simulink library "LopesDevelopmentLibrary"  (R2015b)
settings: Solver=ode45  StartTime=0.0  StopTime=10.0  RelTol=1e-3
values from neighbouring files (symbols this model uses):
  d2r = @(d) d*(pi/180)    [LopesDevelopmentLibrary_LoadParameters.m]
  ts = LopesParams.ts    [LopesDevelopmentLibrary_LoadParameters.m]
undefined symbols (not defined in the file or in its folder): anyParameterChanged, DiscIntNeverNeededParam, gcbh, LHF, LKF, LopesParams, macaddr, mxpcnetworkconfig, mxpcrtudprx, mxpcrtudptx, patientParametersChanged, port, PX, PZ, RHF, RKF, SelectorLOPESInSize, StrideTime_s, Time
undefined symbols (not defined in the file): LopesParamsSendDataArrayLen
libraries: LopesDevelopmentLibrary x288, simulink x98, dspmtrx3 x47, xpciplib x6, xpcnetworkbufferlib x5, dspsigops x4, dspstat3 x3, xpcethernetlib x2, visionstatistics x2, xpcseriallib x2, nmc x1, simulink_extras x1
(part 6 of 12)

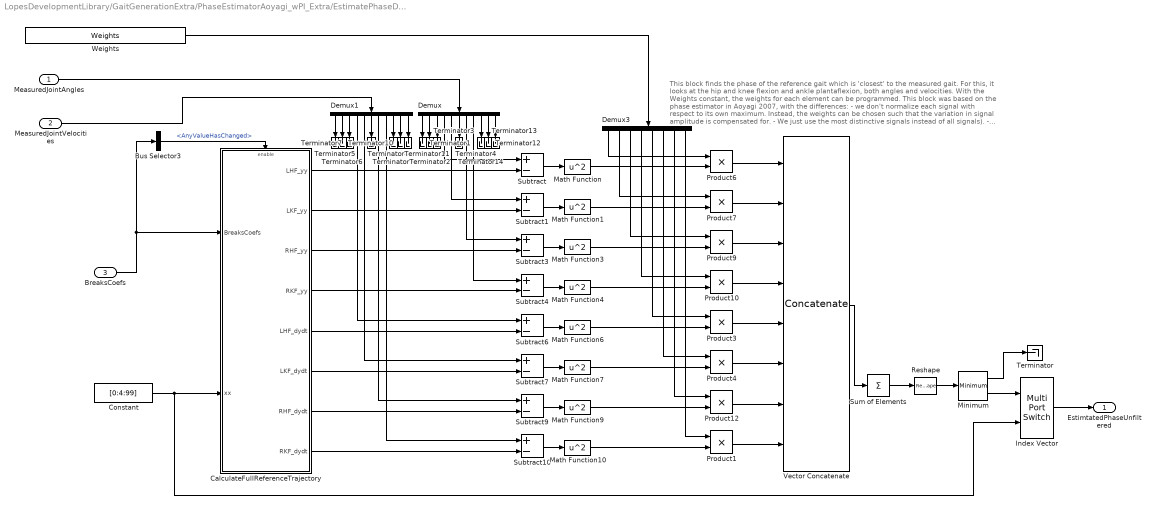
== system LopesDevelopmentLibrary/GaitGenerationExtra/PhaseEstimatorAoyagi_wPI_Extra/EstimatePhaseDirectlyAoyagi ==
  note: This block finds the phase of the reference gait which is 'closest' to the
      | measured gait. For this, it looks at the hip and knee flexion and ankle plantaflexion,
      | both angles and velocities. With the Weights constant, the weights for each element
      | can be programmed.
      | This block was based on the phase estimator in Aoyagi 2007, with the differences:
      | - we don't normalize each signal with respect to its own maximum. Instead, the weights
      | can be chosen such that the variation in signal amplitude is compensated for.
      | - We just use the most distinctive signals instead of all signals).
      | - The phase is expressed in percent  [0,100) instead of [0,1).
  MeasuredJointAngles : Inport
  MeasuredJointVelocities : Inport  Port=2
  BreaksCoefs : Inport  Port=3
  Bus Selector3 : BusSelector  OutputSignals=AnyValueHasChanged
  CalculateFullReferenceTrajectory : Subsystem
  Constant : Constant  Value=[0:4:99]
  Demux : Demux  Outputs=11
  Demux1 : Demux  Outputs=11
  Demux3 : Demux  Outputs=8
  Index Vector : MultiPortSwitch  Inputs=1
  Math Function{,1,3..4,6..7,9..10} (8 alike) : Math  Operator=square  SaturateOnIntegerOverflow=on
  Minimum : dspstat3/Minimum  fcn=Value and Index  reset=None  InputProcessing=Columns as channels (frame based)  indexBase=One  operateOver=Each column  Dimension=1  operation=minimum  roiEnable=off  roiType=Rectangles  roiPortion=Entire ROI  roiOutput=Individual statistics for each ROI  roiFlag=off  roundingMode=Floor  overflowMode=off
  Product{1,3..4,6..7,9..10,12} (8 alike) : Product  RndMeth=Zero
  Reshape : Reshape
  Subtract{,1,3..4,6..7,9..10} (8 alike) : Sum  Inputs=+-
  Sum of Elements : Sum  Inputs=+  CollapseMode=Specified dimension  CollapseDim=2
  Terminator{,1..14} (15 alike) : Terminator
  Vector Concatenate : Concatenate  NumInputs=8  Mode=Multidimensional array  ConcatenateDimension=2
  Weights : Constant  Value=Weights
  EstimtatedPhaseUnfiltered : Outport
  wires:
  Demux3/8 -> Product1/1
  Demux3/7 -> Product12/1
  Demux3/6 -> Product4/1
  Demux3/5 -> Product3/1
  Demux3/4 -> Product10/1
  Demux3/3 -> Product9/1
  Demux3/2 -> Product7/1
  Demux3/1 -> Product6/1
  Bus Selector3/1 -> CalculateFullReferenceTrajectory/Enable  "<AnyValueHasChanged>"
  CalculateFullReferenceTrajectory/8(RKF_dydt) -> Subtract10/2
  CalculateFullReferenceTrajectory/7(RHF_dydt) -> Subtract9/2
  CalculateFullReferenceTrajectory/6(LKF_dydt) -> Subtract7/2
  CalculateFullReferenceTrajectory/5(LHF_dydt) -> Subtract6/2
  CalculateFullReferenceTrajectory/4(RKF_yy) -> Subtract4/2
  CalculateFullReferenceTrajectory/3(RHF_yy) -> Subtract3/2
  CalculateFullReferenceTrajectory/2(LKF_yy) -> Subtract1/2
  CalculateFullReferenceTrajectory/1(LHF_yy) -> Subtract/2
  Reshape/1 -> Minimum/1
  Product1/1 -> Vector Concatenate/8
  Product12/1 -> Vector Concatenate/7
  Product3/1 -> Vector Concatenate/5
  Product4/1 -> Vector Concatenate/6
  Math Function10/1 -> Product1/2
  Math Function9/1 -> Product12/2
  Math Function7/1 -> Product4/2
  Math Function6/1 -> Product3/2
  Demux1/8 -> Subtract10/1
  Demux1/7 -> Subtract9/1
  Demux1/5 -> Subtract7/1
  Demux1/4 -> Subtract6/1
  Subtract10/1 -> Math Function10/1
  Subtract9/1 -> Math Function9/1
  Subtract7/1 -> Math Function7/1
  Subtract6/1 -> Math Function6/1
  MeasuredJointVelocities/1 -> Demux1/1
  Minimum/2 -> Index Vector/1
  Sum of Elements/1 -> Reshape/1
  Vector Concatenate/1 -> Sum of Elements/1
  Product10/1 -> Vector Concatenate/4
  Product9/1 -> Vector Concatenate/3
  Product6/1 -> Vector Concatenate/1
  Product7/1 -> Vector Concatenate/2
  Weights/1 -> Demux3/1
  Math Function4/1 -> Product10/2
  Math Function3/1 -> Product9/2
  Math Function1/1 -> Product7/2
  Math Function/1 -> Product6/2
  Subtract4/1 -> Math Function4/1
  Subtract3/1 -> Math Function3/1
  Subtract1/1 -> Math Function1/1
  Subtract/1 -> Math Function/1
  Demux/8 -> Subtract4/1
  Demux/7 -> Subtract3/1
  Index Vector/1 -> EstimtatedPhaseUnfiltered/1
  BreaksCoefs/1 -> CalculateFullReferenceTrajectory/1(BreaksCoefs), Bus Selector3/1
  MeasuredJointAngles/1 -> Demux/1
  Constant/1 -> CalculateFullReferenceTrajectory/2(xx), Index Vector/2
  Demux/4 -> Subtract/1
  Demux/5 -> Subtract1/1
  Minimum/1 -> Terminator/1
  Demux1/6 -> Terminator8/1
  Demux1/3 -> Terminator7/1
  Demux1/2 -> Terminator6/1
  Demux1/1 -> Terminator5/1
  Demux/1 -> Terminator1/1
  Demux/2 -> Terminator2/1
  Demux/3 -> Terminator3/1
  Demux/6 -> Terminator4/1
  Demux1/9 -> Terminator9/1
  Demux1/10 -> Terminator10/1
  Demux1/11 -> Terminator11/1
  Demux/11 -> Terminator13/1
  Demux/10 -> Terminator12/1
  Demux/9 -> Terminator14/1

== system LopesDevelopmentLibrary/GaitGenerationExtra/PhaseEstimatorAoyagi_wPI_Extra/PhaseFilterAoyagi ==
  note: This filter is based on the filter described in Aoyagi 2007.
      | It differs on the following points:
      | - Range [0,100) %, not [0,1) scale.
      | - Different implementation of wrap around integration (Aoyagi uses a resettable integrator; I use a mod 100)
      | - AoyagiFilterGain should be the same as in the paper (the error is 100 times larger than Aoyagi's, but so is
      |    the range of the integration). I found however that 2.5 for a gain [Aoyagi 2007] is quite low.
      | - In the figure in the paper no saturation is shown, but in the text they tell that there is saturation. I use it
      |    here too (so that phase cannot go backwards and cannot go rise too fast).
  note: "'PI-controller". Makes sure that the phase error will eventually
      | go to zero. Hopefully this will make the system better. However, the integral is
      | limited to -20..20 to prevent problems when a non-walking state is detected.
  EstimatedPhaseUnfiltered : Inport
  ReferenceStrideTime : Inport  Port=2
  ResetHighActive : Inport  Port=3
  x0 : Inport  Port=4
  FinalState : Inport  Port=5
  AoyagiFilterGain : Gain  Gain=AoyagiFilterGain
  CalculateStridesPerSec : Math  Operator=reciprocal  SaturateOnIntegerOverflow=on
  Compare To Constant : simulink/Logic and Bit Operations/Compare To Constant  relop=~=  const=1  OutDataTypeStr=boolean
  Divide : Product  Inputs=/*
  FinalStateFinisher : Subsystem
  Gain : Gain  Gain=3
  Gain1 : Gain  Gain=0.2
  IntegralTimeConstant : Constant  Value=AoyagiIntegralTimeConstant
  Integrator : Integrator  ExternalReset=level  InitialConditionSource=external
  Integrator1 : Integrator  ExternalReset=level  LimitOutput=on  UpperSaturationLimit=20  LowerSaturationLimit=-20
  PhaseWrapper : LopesDevelopmentLibrary/Various/PhaseWrapper
  Product : Product  OutDataTypeStr=double
  Saturation Dynamic : simulink/Discontinuities/Saturation Dynamic  OutMin=[]  OutMax=[]  OutDataTypeStr=Inherit: Same as second input  OutDataType=fixdt(1, 16)  OutScaling=2^-10  DoSatur=off
  Sum : Sum  Inputs=|+-
  Sum1 : Sum  Inputs=++|
  Sum2 : Sum  Inputs=++|
  ToPercentPerSec : Gain  Gain=100
  Wrap_Min50_Plus50 : Subsystem
  EstimatedPhase : Outport
  EstimatedPhaseRate : Outport  Port=2
  wires:
  ResetHighActive/1 -> Integrator1/2, Compare To Constant/1, Integrator/2
  Integrator/1 -> PhaseWrapper/1
  EstimatedPhaseUnfiltered/1 -> Sum/1
  Sum1/1 -> Saturation Dynamic/2
  AoyagiFilterGain/1 -> Sum1/2, Divide/2
  ToPercentPerSec/1 -> Sum2/2, Gain1/1, Gain/1
  PhaseWrapper/1 -> EstimatedPhase/1, Sum/2
  CalculateStridesPerSec/1 -> ToPercentPerSec/1
  Wrap_Min50_Plus50/1(Out) -> AoyagiFilterGain/1
  Sum/1 -> Wrap_Min50_Plus50/1(In)
  ReferenceStrideTime/1 -> CalculateStridesPerSec/1
  Gain1/1 -> Saturation Dynamic/3
  Gain/1 -> Saturation Dynamic/1
  IntegralTimeConstant/1 -> Divide/1
  Divide/1 -> Integrator1/1
  Integrator1/1 -> Sum2/1
  Sum2/1 -> Sum1/1
  x0/1 -> Integrator/3
  Saturation Dynamic/1 -> Product/1
  FinalState/1 -> FinalStateFinisher/2(FinalState)
  FinalStateFinisher/1(PhasePercRateOut) -> EstimatedPhaseRate/1, Integrator/1
  Compare To Constant/1 -> Product/2
  Product/1 -> FinalStateFinisher/1(PhasePercRate)

== system LopesDevelopmentLibrary/GaitGenerationExtra/VelocityHold/RateLimiterWithReset ==
  note: If EnableRateLimit is nonzero, the rate of u is limited.
      | If EnableRateLimit is zero, the value is set to resetValue instantly
      | Note, I used 1e100 instead of inf because inf is not suppported by TwinCAT.
  u : Inport
  ResetRateLimit : Inport  Port=2
  resetValue : Inport  Port=3
  FallingSlewRate : Constant  Value=FallingSlewRate
  FallingSlewRateDisabled : Constant  Value=-1e100
  Rate Limiter Dynamic : simulink/Discontinuities/Rate Limiter Dynamic
  RisingSlewRate : Constant  Value=RisingSlewRate
  RisingSlewRateDisabled : Constant  Value=1e100
  Switch : Switch  Criteria=u2 ~= 0
  Switch1 : Switch  Criteria=u2 ~= 0
  Switch2 : Switch  Criteria=u2 ~= 0
  y : Outport
  wires:
  FallingSlewRateDisabled/1 -> Switch1/1
  Switch/1 -> Rate Limiter Dynamic/1
  RisingSlewRate/1 -> Switch/3
  RisingSlewRateDisabled/1 -> Switch/1
  ResetRateLimit/1 -> Switch2/2, Switch1/2, Switch/2
  Rate Limiter Dynamic/1 -> y/1
  resetValue/1 -> Switch2/1
  Switch1/1 -> Rate Limiter Dynamic/3
  FallingSlewRate/1 -> Switch1/3
  u/1 -> Switch2/3
  Switch2/1 -> Rate Limiter Dynamic/2

== system LopesDevelopmentLibrary/GaitPhaseDetection/Gait Phase Detection with Wrapper/Data selection ==
  Cart_pos : Inport
  Treadmill : Inport  Port=2
  Angle_l : Subsystem
  Angle_r : Subsystem
  Selector : Selector  InputPortWidth=21  IndexOptions=Index vector (dialog)  Indices=[11]  OutputSizes=1
  Selector1 : Selector  InputPortWidth=21  IndexOptions=Index vector (dialog)  Indices=[20]  OutputSizes=1
  Selector10 : Selector  InputPortWidth=21  IndexOptions=Index vector (dialog)  Indices=[16 17 18]  OutputSizes=1
  Selector11 : Selector  InputPortWidth=21  IndexOptions=Index vector (dialog)  Indices=[13 14 15]  OutputSizes=1
  Selector2 : Selector  InputPortWidth=21  IndexOptions=Index vector (dialog)  Indices=[19]  OutputSizes=1
  Selector3 : Selector  InputPortWidth=21  IndexOptions=Index vector (dialog)  Indices=[10]  OutputSizes=1
  Selector4 : Selector  InputPortWidth=7  IndexOptions=Index vector (dialog)  Indices=[2]  OutputSizes=1
  Selector5 : Selector  InputPortWidth=21  IndexOptions=Index vector (dialog)  Indices=[10 11 12]  OutputSizes=1
  Selector6 : Selector  InputPortWidth=21  IndexOptions=Index vector (dialog)  Indices=[7 8 9]  OutputSizes=1
  Selector7 : Selector  InputPortWidth=21  IndexOptions=Index vector (dialog)  Indices=[4 5 6]  OutputSizes=1
  Selector9 : Selector  InputPortWidth=21  IndexOptions=Index vector (dialog)  Indices=[19 20 21]  OutputSizes=1
  ankle_y_l : Outport
  ankle_x_l : Outport  Port=2
  angle_knee_l : Outport  Port=3
  ankle_y_r : Outport  Port=4
  ankle_x_r : Outport  Port=5
  angle_knee_r : Outport  Port=6
  Treadmill speed : Outport  Port=7
  wires:
  Selector2/1 -> ankle_x_r/1
  Treadmill/1 -> Selector4/1
  Selector3/1 -> ankle_x_l/1
  Selector4/1 -> Treadmill speed/1
  Selector1/1 -> ankle_y_r/1
  Selector/1 -> ankle_y_l/1
  Cart_pos/1 -> Selector5/1, Selector10/1, Selector11/1, Selector9/1, Selector7/1, Selector6/1, Selector2/1, Selector1/1, Selector3/1, Selector/1
  Selector5/1 -> Angle_l/1(ankle)
  Selector6/1 -> Angle_l/2(knee)
  Selector7/1 -> Angle_l/3(hip)
  Selector10/1 -> Angle_r/2(knee)
  Selector9/1 -> Angle_r/1(ankle)
  Selector11/1 -> Angle_r/3(hip)
  Angle_l/1(angle_l) -> angle_knee_l/1
  Angle_r/1(angle_r) -> angle_knee_r/1

== system LopesDevelopmentLibrary/GaitPhaseDetection/Gait Phase Detection with Wrapper/LeftLegWalking ==
  note: Right foot detection
      | 1 = stance phase
      | 2 = swing phase
  ankle_y_r_dot : Inport
  ankle_x_r_dot : Inport  Port=2
  knee_angle_dot : Inport  Port=3
  belt_speed : Inport  Port=4
  Add2 : Sum  OutDataTypeStr=double
  Heel strike detection : Subsystem
  Heel strike_safety : Subsystem
  Logical Operator2 : Logic  Operator=OR  AllPortsSameDT=off  OutDataTypeStr=boolean
  Sample and Hold2 : dspsigops/Sample and Hold  trig=Rising edge  initCond=1  latchinput=off
  Toe-off detection : Subsystem
  Left : Outport  OutDataTypeStr=double
  wires:
  knee_angle_dot/1 -> Toe-off detection/2(knee_angle_dot)
  Heel strike_safety/1(Heel_strike_safety) -> Logical Operator2/2
  belt_speed/1 -> Heel strike_safety/2(belt_speed)
  Toe-off detection/1(Toe_off) -> Add2/2
  Heel strike detection/1(Heel_strike) -> Logical Operator2/1
  ankle_y_r_dot/1 -> Heel strike detection/1(ankle_y_dot)  "ankle_y_dot"
  ankle_x_r_dot/1 -> Toe-off detection/1(ankle_x_dot), Heel strike detection/2(ankle_x_dot), Heel strike_safety/1(ankle_x_dot)  "ankle_x_dot"
  Add2/1 -> Sample and Hold2/1, Sample and Hold2/Trigger
  Logical Operator2/1 -> Add2/1
  Sample and Hold2/1 -> Left/1

== system LopesDevelopmentLibrary/GaitPhaseDetection/Gait Phase Detection with Wrapper/No speed detection ==
  note: If the treadmill velocity is above 0.05 and 250 ms have passed
      | since the start of the simulation, gait initiation can be detected using the "normal" method
      | If Velocity of treadmill is too low, the COP is used to estimate swing/stance
  note: Detection
      | 1 = stance phase
      | 2 = swing phase
  note: If COP is 5x closer to foot 1 than foot 2, foot 2 is assumed to be in swing
  curVel : Inport
  CartesianPositions : Inport  Port=2
  Treadmill : Inport  Port=3
  "   " : MinMax
  "        " : simulink/Discrete/Tapped Delay  vinit=0  samptime=-1  NumDelays=250  DelayOrder=Oldest  includeCurrent=off
  Ankle_L_XZ : Selector  InputPortWidth=21  IndexOptions=Index vector (dialog)  Indices=[10 12]  OutputSizes=1
  Ankle_R_XZ : Selector  InputPortWidth=21  IndexOptions=Index vector (dialog)  Indices=[19 21]  OutputSizes=1
  COP_XZ : Selector  InputPortWidth=7  IndexOptions=Index vector (dialog)  Indices=[5 6]  OutputSizes=1
  Compare To Constant : simulink/Logic and Bit Operations/Compare To Constant  relop=<=  const=0.2  OutDataTypeStr=boolean
  Compare To Constant1 : simulink/Logic and Bit Operations/Compare To Constant  relop=>=  const=0.05  OutDataTypeStr=uint8  ZeroCross=off
  Compare To Constant2 : simulink/Logic and Bit Operations/Compare To Constant  relop=<=  const=0.2  OutDataTypeStr=boolean
  Constant : Constant  Value=2
  Constant1 : Constant
  Data Type Conversion : DataTypeConversion
  DistLeft : Fcn  Expr=((u(1) - u(3))^2 + (u(2) - u(4))^2)^0.5
  DistRight : Fcn  Expr=((u(1) - u(3))^2 + (u(2) - u(4))^2)^0.5
  Divide : Product  Inputs=*/
  Divide1 : Product  Inputs=*/
  LeftFoot : Switch  Criteria=u2 > Threshold
  Mux : Mux  Inputs=2
  Mux1 : Mux  Inputs=2
  RightFoot : Switch  Criteria=u2 > Threshold
  gaitSwitch : Outport
  Left : Outport  Port=2
  Right : Outport  Port=3
  wires:
  Compare To Constant1/1 -> Data Type Conversion/1
  curVel/1 -> "        "/1
  Data Type Conversion/1 -> gaitSwitch/1
  "        "/1 -> "   "/1
  "   "/1 -> Compare To Constant1/1
  CartesianPositions/1 -> Ankle_R_XZ/1, Ankle_L_XZ/1
  Treadmill/1 -> COP_XZ/1
  Mux/1 -> DistLeft/1
  Ankle_L_XZ/1 -> Mux/1
  COP_XZ/1 -> Mux1/2, Mux/2
  Ankle_R_XZ/1 -> Mux1/1
  Mux1/1 -> DistRight/1
  DistLeft/1 -> Divide1/2, Divide/1
  DistRight/1 -> Divide/2, Divide1/1
  Divide/1 -> Compare To Constant/1
  Divide1/1 -> Compare To Constant2/1
  Compare To Constant/1 -> RightFoot/2
  Compare To Constant2/1 -> LeftFoot/2
  Constant/1 -> LeftFoot/1, RightFoot/1
  Constant1/1 -> RightFoot/3, LeftFoot/3
  LeftFoot/1 -> Left/1
  RightFoot/1 -> Right/1

== system LopesDevelopmentLibrary/GaitPhaseDetection/Gait Phase Detection with Wrapper/Phase_selection ==
  LeftWalking : Inport
  RightWalking : Inport  Port=2
  Gait_switch : Inport  Port=3
  ankle_x_l : Inport  Port=4
  ankle_x_r : Inport  Port=5
  LeftStop : Inport  Port=6
  RightStop : Inport  Port=7
  Delay : Delay  DelayLength=1  InitialCondition=0
  MATLAB Function : MATLAB Function  TreatAsAtomicUnit=on
  Phase : Outport
  wires:
  MATLAB Function/1(y) -> Delay/1, Phase/1
  Delay/1 -> MATLAB Function/8(prev)
  LeftWalking/1 -> MATLAB Function/1(leftWalking)
  RightWalking/1 -> MATLAB Function/2(rightWalking)
  Gait_switch/1 -> MATLAB Function/5(switchSignal)
  ankle_x_l/1 -> MATLAB Function/6(left_x)
  ankle_x_r/1 -> MATLAB Function/7(right_x)
  LeftStop/1 -> MATLAB Function/3(leftStop)
  RightStop/1 -> MATLAB Function/4(rightStop)

== system LopesDevelopmentLibrary/GaitPhaseDetection/Gait Phase Detection with Wrapper/RightLegWalking ==
  note: Right foot detection
      | 1 = stance phase
      | 2 = swing phase
  ankle_y_r_dot : Inport
  ankle_x_r_dot : Inport  Port=2
  knee_angle_dot : Inport  Port=3
  belt_speed : Inport  Port=4
  Add2 : Sum  OutDataTypeStr=double
  Heel strike detection : Subsystem
  Heel strike_safety : Subsystem
  Logical Operator2 : Logic  Operator=OR  AllPortsSameDT=off  OutDataTypeStr=boolean
  Sample and Hold2 : dspsigops/Sample and Hold  trig=Rising edge  initCond=1  latchinput=off
  Toe-off detection : Subsystem
  right : Outport  OutDataTypeStr=double
  wires:
  Sample and Hold2/1 -> right/1
  Logical Operator2/1 -> Add2/1
  Add2/1 -> Sample and Hold2/Trigger, Sample and Hold2/1
  ankle_x_r_dot/1 -> Heel strike_safety/1(ankle_x_dot), Heel strike detection/2(ankle_x_dot), Toe-off detection/1(ankle_x_dot)  "ankle_x_dot"
  ankle_y_r_dot/1 -> Heel strike detection/1(ankle_y_dot)  "ankle_y_dot"
  Heel strike detection/1(Heel_strike) -> Logical Operator2/1
  Toe-off detection/1(Toe_off) -> Add2/2
  belt_speed/1 -> Heel strike_safety/2(belt_speed)
  Heel strike_safety/1(Heel_strike_safety) -> Logical Operator2/2
  knee_angle_dot/1 -> Toe-off detection/2(knee_angle_dot)

== system LopesDevelopmentLibrary/GaitPhaseDetection/Gait Phase Detection with Wrapper/Smart derivative ==
  note: The filter order is regulated by the belt speed to promote
      | efficiency and accuracy
  ankle_y_l : Inport
  ankle_x_l : Inport  Port=2
  angle_knee_l : Inport  Port=3
  ankle_y_r : Inport  Port=4
  ankle_x_r : Inport  Port=5
  angle_knee_r : Inport  Port=6
  treadmill speed : Inport  Port=7
  Filtered derivative : Subsystem
  Filtered derivative1 : Subsystem
  Filtered derivative2 : Subsystem
  Filtered derivative3 : Subsystem
  Filtered derivative4 : Subsystem
  Filtered derivative5 : Subsystem
  belt_speed to cut-off : Subsystem
  ankle_y_l_dot : Outport
  ankle_x_l_dot : Outport  Port=2
  angle_knee_l_dot : Outport  Port=3
  ankle_y_r_dot : Outport  Port=4
  ankle_x_r_dot : Outport  Port=5
  angle_knee_r_dot : Outport  Port=6
  wires:
  ankle_y_l/1 -> Filtered derivative/1(x)
  Filtered derivative/1(x_dot) -> ankle_y_l_dot/1
  ankle_x_l/1 -> Filtered derivative1/1(x)
  angle_knee_l/1 -> Filtered derivative2/1(x)
  ankle_y_r/1 -> Filtered derivative3/1(x)
  ankle_x_r/1 -> Filtered derivative4/1(x)
  angle_knee_r/1 -> Filtered derivative5/1(x)
  Filtered derivative2/1(x_dot) -> angle_knee_l_dot/1
  Filtered derivative3/1(x_dot) -> ankle_y_r_dot/1
  Filtered derivative4/1(x_dot) -> ankle_x_r_dot/1
  Filtered derivative5/1(x_dot) -> angle_knee_r_dot/1
  belt_speed to cut-off/1(cut-off (hz)) -> Filtered derivative5/2(cut-off (hz)), Filtered derivative4/2(cut-off (hz)), Filtered derivative3/2(cut-off (hz)), Filtered derivative2/2(cut-off (hz)), Filtered derivative1/2(cut-off (hz)), Filtered derivative/2(cut-off (hz))
  treadmill speed/1 -> belt_speed to cut-off/1(belt speed)
  Filtered derivative1/1(x_dot) -> ankle_x_l_dot/1

== system LopesDevelopmentLibrary/GaitPhaseDetection/Gait Phase detection/Data selection ==
  Cart_pos : Inport
  Treadmill : Inport  Port=2
  Angle_l : Subsystem
  Angle_r : Subsystem
  Selector : Selector  InputPortWidth=21  IndexOptions=Index vector (dialog)  Indices=[11]  OutputSizes=1
  Selector1 : Selector  InputPortWidth=21  IndexOptions=Index vector (dialog)  Indices=[20]  OutputSizes=1
  Selector10 : Selector  InputPortWidth=21  IndexOptions=Index vector (dialog)  Indices=[16 17 18]  OutputSizes=1
  Selector11 : Selector  InputPortWidth=21  IndexOptions=Index vector (dialog)  Indices=[13 14 15]  OutputSizes=1
  Selector2 : Selector  InputPortWidth=21  IndexOptions=Index vector (dialog)  Indices=[19]  OutputSizes=1
  Selector3 : Selector  InputPortWidth=21  IndexOptions=Index vector (dialog)  Indices=[10]  OutputSizes=1
  Selector4 : Selector  InputPortWidth=7  IndexOptions=Index vector (dialog)  Indices=[2]  OutputSizes=1
  Selector5 : Selector  InputPortWidth=21  IndexOptions=Index vector (dialog)  Indices=[10 11 12]  OutputSizes=1
  Selector6 : Selector  InputPortWidth=21  IndexOptions=Index vector (dialog)  Indices=[7 8 9]  OutputSizes=1
  Selector7 : Selector  InputPortWidth=21  IndexOptions=Index vector (dialog)  Indices=[4 5 6]  OutputSizes=1
  Selector9 : Selector  InputPortWidth=21  IndexOptions=Index vector (dialog)  Indices=[19 20 21]  OutputSizes=1
  ankle_y_l : Outport
  ankle_x_l : Outport  Port=2
  angle_knee_l : Outport  Port=3
  ankle_y_r : Outport  Port=4
  ankle_x_r : Outport  Port=5
  angle_knee_r : Outport  Port=6
  Treadmill speed : Outport  Port=7
  wires:
  Angle_r/1(angle_r) -> angle_knee_r/1
  Angle_l/1(angle_l) -> angle_knee_l/1
  Selector11/1 -> Angle_r/3(hip)
  Selector9/1 -> Angle_r/1(ankle)
  Selector10/1 -> Angle_r/2(knee)
  Selector7/1 -> Angle_l/3(hip)
  Selector6/1 -> Angle_l/2(knee)
  Selector5/1 -> Angle_l/1(ankle)
  Cart_pos/1 -> Selector/1, Selector3/1, Selector1/1, Selector2/1, Selector6/1, Selector7/1, Selector9/1, Selector11/1, Selector10/1, Selector5/1
  Selector/1 -> ankle_y_l/1
  Selector1/1 -> ankle_y_r/1
  Selector4/1 -> Treadmill speed/1
  Selector3/1 -> ankle_x_l/1
  Treadmill/1 -> Selector4/1
  Selector2/1 -> ankle_x_r/1

== system LopesDevelopmentLibrary/GaitPhaseDetection/Gait Phase detection/LeftLeg ==
  note: Left foot detection
      | 1 = stance phase
      | 2 = swing phase
  ankle_y_l_dot : Inport
  ankle_x_l_dot : Inport  Port=2
  knee_theta_l_dot : Inport  Port=3
  belt_speed : Inport  Port=4
  Add1 : Sum
  Heel strike detection : Subsystem
  Heel strike_safety : Subsystem
  Logical Operator1 : Logic  Operator=OR  AllPortsSameDT=off  OutDataTypeStr=boolean
  Sample and Hold1 : dspsigops/Sample and Hold  trig=Rising edge  initCond=1  latchinput=off
  Toe-off detection : Subsystem
  left : Outport
  wires:
  knee_theta_l_dot/1 -> Toe-off detection/2(knee_angle_dot)
  Heel strike_safety/1(Heel_strike_safety) -> Logical Operator1/2
  belt_speed/1 -> Heel strike_safety/2(belt_speed)
  Toe-off detection/1(Toe_off) -> Add1/2
  Heel strike detection/1(Heel_strike) -> Logical Operator1/1
  ankle_y_l_dot/1 -> Heel strike detection/1(ankle_y_dot)  "ankle_y_dot"
  ankle_x_l_dot/1 -> Heel strike detection/2(ankle_x_dot), Toe-off detection/1(ankle_x_dot), Heel strike_safety/1(ankle_x_dot)  "ankle_x_dot"
  Add1/1 -> Sample and Hold1/1, Sample and Hold1/Trigger
  Logical Operator1/1 -> Add1/1
  Sample and Hold1/1 -> left/1

== system LopesDevelopmentLibrary/GaitPhaseDetection/Gait Phase detection/No speed detection ==
  note: If the treadmill velocity is above 0.05 and 1.5 seconds have passed
      | since the start of the simulation, gait initiation can be detected
  curVel : Inport
  "   " : MinMax
  "        " : simulink/Discrete/Tapped Delay  vinit=0  samptime=-1  NumDelays=1500  DelayOrder=Oldest  includeCurrent=off
  Compare To Constant1 : simulink/Logic and Bit Operations/Compare To Constant  relop=>=  const=0.05  OutDataTypeStr=uint8  ZeroCross=off
  Data Type Conversion : DataTypeConversion
  gaitSwitch : Outport
  wires:
  "   "/1 -> Compare To Constant1/1
  "        "/1 -> "   "/1
  Data Type Conversion/1 -> gaitSwitch/1
  curVel/1 -> "        "/1
  Compare To Constant1/1 -> Data Type Conversion/1

== system LopesDevelopmentLibrary/GaitPhaseDetection/Gait Phase detection/Phase_selection ==
  Left : Inport
  Right : Inport  Port=2
  Gait_switch : Inport  Port=3
  ankle_x_l : Inport  Port=4
  ankle_x_r : Inport  Port=5
  MATLAB Function : MATLAB Function  TreatAsAtomicUnit=on
  Phase : Outport
  wires:
  ankle_x_r/1 -> MATLAB Function/5(right_x)
  ankle_x_l/1 -> MATLAB Function/4(left_x)
  Gait_switch/1 -> MATLAB Function/3(belt)
  Right/1 -> MATLAB Function/2(right)
  Left/1 -> MATLAB Function/1(left)
  MATLAB Function/1(y) -> Phase/1

== system LopesDevelopmentLibrary/GaitPhaseDetection/Gait Phase detection/RightLeg ==
  note: Right foot detection
      | 1 = stance phase
      | 2 = swing phase
  ankle_y_r_dot : Inport
  ankle_x_r_dot : Inport  Port=2
  knee_angle_dot : Inport  Port=3
  belt_speed : Inport  Port=4
  Add2 : Sum
  Heel strike detection1 : Subsystem
  Heel strike_safety1 : Subsystem
  Logical Operator2 : Logic  Operator=OR  AllPortsSameDT=off  OutDataTypeStr=boolean
  Sample and Hold2 : dspsigops/Sample and Hold  trig=Rising edge  initCond=1  latchinput=off
  Toe-off detection1 : Subsystem
  right : Outport
  wires:
  knee_angle_dot/1 -> Toe-off detection1/2(knee_angle_dot)
  Heel strike_safety1/1(Heel_strike_safety) -> Logical Operator2/2
  belt_speed/1 -> Heel strike_safety1/2(belt_speed)
  Toe-off detection1/1(Toe_off) -> Add2/2
  Heel strike detection1/1(Heel_strike) -> Logical Operator2/1
  ankle_y_r_dot/1 -> Heel strike detection1/1(ankle_y_dot)  "ankle_y_dot"
  ankle_x_r_dot/1 -> Heel strike_safety1/1(ankle_x_dot), Toe-off detection1/1(ankle_x_dot), Heel strike detection1/2(ankle_x_dot)  "ankle_x_dot"
  Add2/1 -> Sample and Hold2/1, Sample and Hold2/Trigger
  Logical Operator2/1 -> Add2/1
  Sample and Hold2/1 -> right/1

== system LopesDevelopmentLibrary/GaitPhaseDetection/Gait Phase detection/Smart derivative ==
  note: The filter order is regulated by the belt speed to promote
      | efficiency and accuracy
  ankle_y_l : Inport
  ankle_x_l : Inport  Port=2
  angle_knee_l : Inport  Port=3
  ankle_y_r : Inport  Port=4
  ankle_x_r : Inport  Port=5
  angle_knee_r : Inport  Port=6
  treadmill speed : Inport  Port=7
  Filtered derivative : Subsystem
  Filtered derivative1 : Subsystem
  Filtered derivative2 : Subsystem
  Filtered derivative3 : Subsystem
  Filtered derivative4 : Subsystem
  Filtered derivative5 : Subsystem
  belt_speed to cut-off : Subsystem
  ankle_y_l_dot : Outport
  ankle_x_l_dot : Outport  Port=2
  angle_knee_l_dot : Outport  Port=3
  ankle_y_r_dot : Outport  Port=4
  ankle_x_r_dot : Outport  Port=5
  angle_knee_r_dot : Outport  Port=6
  wires:
  Filtered derivative1/1(x_dot) -> ankle_x_l_dot/1
  treadmill speed/1 -> belt_speed to cut-off/1(belt speed)
  belt_speed to cut-off/1(cut-off (hz)) -> Filtered derivative5/2(cut-off (hz)), Filtered derivative4/2(cut-off (hz)), Filtered derivative3/2(cut-off (hz)), Filtered derivative2/2(cut-off (hz)), Filtered derivative1/2(cut-off (hz)), Filtered derivative/2(cut-off (hz))
  Filtered derivative5/1(x_dot) -> angle_knee_r_dot/1
  Filtered derivative4/1(x_dot) -> ankle_x_r_dot/1
  Filtered derivative3/1(x_dot) -> ankle_y_r_dot/1
  Filtered derivative2/1(x_dot) -> angle_knee_l_dot/1
  angle_knee_r/1 -> Filtered derivative5/1(x)
  ankle_x_r/1 -> Filtered derivative4/1(x)
  ankle_y_r/1 -> Filtered derivative3/1(x)
  angle_knee_l/1 -> Filtered derivative2/1(x)
  ankle_x_l/1 -> Filtered derivative1/1(x)
  Filtered derivative/1(x_dot) -> ankle_y_l_dot/1
  ankle_y_l/1 -> Filtered derivative/1(x)

== system LopesDevelopmentLibrary/Mindwalker/Mindwalker_Lopes_Conversion/CalculateForceOnTorso ==
  MW_SpringPositions : Inport
  MW_SpringVelocities : Inport  Port=2
  MW_SpringStiffness : Inport  Port=3
  MW_BiasForces : Inport  Port=4
  Lopes_ModelPos : Inport  Port=5
  Lopes_ModelVel : Inport  Port=6
  Inertia : Inport  Port=7
  Add : Sum  Inputs=1
  CalculateDampingTerm : Subsystem
  GetLHFandRHF : Selector  InputPortWidth=11  IndexOptions=Index vector (dialog)  Indices=[4,7]  OutputSizes=1
  GetLHFandRHF1 : Selector  InputPortWidth=8  IndexOptions=Index vector (dialog)  Indices=[4,7]  OutputSizes=1
  GetLHFandRHF2 : Selector  InputPortWidth=11  IndexOptions=Index vector (dialog)  Indices=[4,7]  OutputSizes=1
  GetLHFandRHF3 : Selector  InputPortWidth=8  IndexOptions=Index vector (dialog)  Indices=[4,7]  OutputSizes=1
  GetLHFandRHF4 : Selector  InputPortWidth=6  IndexOptions=Index vector (dialog)  Indices=[2,5]  OutputSizes=1
  GetLHFandRHF5 : Selector  InputPortWidth=6  IndexOptions=Index vector (dialog)  Indices=[2,5]  OutputSizes=1
  Mux : Mux  Inputs=3
  Product : Product  RndMeth=Zero
  Product1 : Product  RndMeth=Zero
  Subtract : Sum  Inputs=+-
  Subtract1 : Sum  Inputs=+-
  Unary Minus : UnaryMinus
  ForceOnTorso : Outport
  wires:
  Add/1 -> ForceOnTorso/1  "TotalForceOnTorso"
  MW_SpringVelocities/1 -> GetLHFandRHF3/1
  Inertia/1 -> CalculateDampingTerm/2(Inertia)
  MW_SpringStiffness/1 -> GetLHFandRHF4/1
  MW_BiasForces/1 -> GetLHFandRHF5/1
  Lopes_ModelPos/1 -> GetLHFandRHF/1
  MW_SpringPositions/1 -> GetLHFandRHF1/1
  GetLHFandRHF5/1 -> Unary Minus/1
  Unary Minus/1 -> Mux/3
  Mux/1 -> Add/1
  GetLHFandRHF3/1 -> Subtract1/1
  GetLHFandRHF2/1 -> Subtract1/2
  GetLHFandRHF1/1 -> Subtract/1
  GetLHFandRHF/1 -> Subtract/2
  CalculateDampingTerm/1(Damping) -> Product1/1
  Subtract/1 -> Product/2
  GetLHFandRHF4/1 -> CalculateDampingTerm/1(Stiffness), Product/1
  Subtract1/1 -> Product1/2
  Lopes_ModelVel/1 -> GetLHFandRHF2/1
  Product/1 -> Mux/1
  Product1/1 -> Mux/2

== system LopesDevelopmentLibrary/Mindwalker/Mindwalker_Lopes_Conversion/LopesToMWPosition ==
  note: This block works for angles as well as velocities
  note: Lopes_Joints:
      | PX (=0)
      | PZ (=0)
      | LHA
      | LHF (absolute; actually Left Thigh Angle)
      | LKF
      | RHA
      | RHF
      | RKF
      | ----
      | PY
      | PAX
      | POB
  note: MW_Joints:
      | LHA
      | LHFR (Left Hip Flexion, Relative)
      | LKF
      | RHA
      | RHFR (Right HIp Flexion, Relative)
      | RKF
      | -----
      | TF = TorsoFlexion (shouldes forward is positive)
      | TOB = TorsoObliquity (shoulders to right is positive)
  Lopes_Joints : Inport
  TorsoValue : Inport  Port=2
  Add : Sum
  Add1 : Sum
  Demux : Demux  Outputs=11
  Mux : Mux  Inputs=8
  Terminator{,1..4} (5 alike) : Terminator
  Zero : Constant  Value=0
  MW_Joints : Outport
  wires:
  Demux/7 -> Add1/1
  Add1/1 -> Mux/5  "RHFR"
  Demux/4 -> Add/1
  Add/1 -> Mux/2  "LHFR"
  Demux/11 -> Terminator4/1  "POB"
  Demux/10 -> Terminator3/1  "PAX"
  Demux/9 -> Terminator2/1  "PY"
  Zero/1 -> Mux/8  "TOB"
  Demux/8 -> Mux/6  "RKF"
  Demux/6 -> Mux/4  "RHA"
  Demux/5 -> Mux/3  "LKF"
  Demux/3 -> Mux/1  "LHA"
  Demux/2 -> Terminator1/1  "PZ"
  Demux/1 -> Terminator/1  "PX"
  TorsoValue/1 -> Mux/7, Add/2, Add1/2  "TF"
  Lopes_Joints/1 -> Demux/1
  Mux/1 -> MW_Joints/1

== system LopesDevelopmentLibrary/Mindwalker/Mindwalker_Lopes_Conversion/LopesToMWVelocity ==
  note: MW_Joints:
      | LHA
      | LHFR (Left Hip Flexion, Relative)
      | LKF
      | RHA
      | RHFR (Right HIp Flexion, Relative)
      | RKF
      | -----
      | TF = TorsoFlexion (shouldes forward is positive)
      | TOB = TorsoObliquity (shoulders to right is positive)
  note: Lopes_Joints:
      | PX (=0)
      | PZ (=0)
      | LHA
      | LHF (absolute; actually Left Thigh Angle)
      | LKF
      | RHA
      | RHF
      | RKF
      | ----
      | PY
      | PAX
      | POB
  note: This block works for angles as well as velocities
  Lopes_Joints : Inport
  TorsoValue : Inport  Port=2
  Add : Sum
  Add1 : Sum
  Demux : Demux  Outputs=11
  Mux : Mux  Inputs=8
  Terminator{,1..4} (5 alike) : Terminator
  Zero : Constant  Value=0
  MW_Joints : Outport
  wires:
  Mux/1 -> MW_Joints/1
  Lopes_Joints/1 -> Demux/1
  TorsoValue/1 -> Add1/2, Add/2, Mux/7  "TF"
  Demux/1 -> Terminator/1  "PX"
  Demux/2 -> Terminator1/1  "PZ"
  Demux/3 -> Mux/1  "LHA"
  Demux/5 -> Mux/3  "LKF"
  Demux/6 -> Mux/4  "RHA"
  Demux/8 -> Mux/6  "RKF"
  Zero/1 -> Mux/8  "TOB"
  Demux/9 -> Terminator2/1  "PY"
  Demux/10 -> Terminator3/1  "PAX"
  Demux/11 -> Terminator4/1  "POB"
  Add/1 -> Mux/2  "LHFR"
  Demux/4 -> Add/1
  Add1/1 -> Mux/5  "RHFR"
  Demux/7 -> Add1/1

== system LopesDevelopmentLibrary/Mindwalker/Mindwalker_Lopes_Conversion/MWToLopesPosition ==
  note: RelativeJoints:
      | LHA
      | LHFR (Left Hip Flexion, Relative)
      | LKF
      | RHA
      | RHFR (Right HIp Flexion, Relative)
      | RKF
  note: AbsoluteJoints:
      | PX (=0)
      | PZ (=0)
      | LHA
      | LHF (absolute; actually Left Thigh Angle)
      | LKF
      | RHA
      | RHF
      | RKF
  note: This block works for angles as well as velocities
  RelativeJoints : Inport
  TorsoValue : Inport  Port=2
  Demux : Demux  Outputs=6
  Mux : Mux  Inputs=8
  Subtract : Sum  Inputs=+-
  Subtract1 : Sum  Inputs=+-
  Zero : Constant  Value=0
  Zero1 : Constant  Value=0
  AbsoluteJoints : Outport
  wires:
  Demux/4 -> Mux/6  "RHA"
  Demux/3 -> Mux/5  "LKF"
  Mux/1 -> AbsoluteJoints/1
  Demux/6 -> Mux/8  "RKF"
  Zero/1 -> Mux/1  "PX"
  RelativeJoints/1 -> Demux/1
  Demux/2 -> Subtract/1
  Zero1/1 -> Mux/2  "PZ"
  Demux/1 -> Mux/3  "LHA"
  Subtract/1 -> Mux/4  "LHF"
  TorsoValue/1 -> Subtract1/2, Subtract/2
  Demux/5 -> Subtract1/1
  Subtract1/1 -> Mux/7  "RHF"

== system LopesDevelopmentLibrary/Mindwalker/Mindwalker_Lopes_Conversion/MWToLopesVelocity ==
  note: This block works for angles as well as velocities
  note: AbsoluteJoints:
      | PX (=0)
      | PZ (=0)
      | LHA
      | LHF (absolute; actually Left Thigh Angle)
      | LKF
      | RHA
      | RHF
      | RKF
  note: RelativeJoints:
      | LHA
      | LHFR (Left Hip Flexion, Relative)
      | LKF
      | RHA
      | RHFR (Right HIp Flexion, Relative)
      | RKF
  RelativeJoints : Inport
  TorsoValue : Inport  Port=2
  Demux : Demux  Outputs=6
  Mux : Mux  Inputs=8
  Subtract : Sum  Inputs=+-
  Subtract1 : Sum  Inputs=+-
  Zero : Constant  Value=0
  Zero1 : Constant  Value=0
  AbsoluteJoints : Outport
  wires:
  Subtract1/1 -> Mux/7  "RHF"
  Demux/5 -> Subtract1/1
  TorsoValue/1 -> Subtract/2, Subtract1/2
  Subtract/1 -> Mux/4  "LHF"
  Demux/1 -> Mux/3  "LHA"
  Zero1/1 -> Mux/2  "PZ"
  Demux/2 -> Subtract/1
  RelativeJoints/1 -> Demux/1
  Zero/1 -> Mux/1  "PX"
  Demux/6 -> Mux/8  "RKF"
  Mux/1 -> AbsoluteJoints/1
  Demux/3 -> Mux/5  "LKF"
  Demux/4 -> Mux/6  "RHA"

== system LopesDevelopmentLibrary/Mindwalker/Mindwalker_Lopes_Conversion/TorsoDynamics ==
  note: This block calculates the torso angle and velocity. Bending forward is positive.
      | The UnitDelay is to make sure we don't get algebraic loops.
  Force : Inport
  Inertia : Inport  Port=2
  Add : Sum
  CalcTorsoAcc : Product  Inputs=*/
  CalcTorsoFlexion : Integrator
  CalcTorsoVelocity : Integrator
  EndStops : Subsystem
  Sum : Sum  Inputs=|++
  TorsoSpring : Subsystem
  Unit Delay : UnitDelay  SampleTime=-1
  TorsoFlexion : Outport
  TorsoFlexionVelocity : Outport  Port=2
  wires:
  Add/1 -> Sum/2
  TorsoSpring/1(Force) -> Add/2
  EndStops/1(EndstopForce) -> Add/1
  Force/1 -> Sum/1
  CalcTorsoFlexion/1 -> TorsoSpring/1(TorsoPos), EndStops/1(TorsoPos), TorsoFlexion/1
  CalcTorsoVelocity/1 -> CalcTorsoFlexion/1, TorsoSpring/2(TorsoVel), EndStops/2(TorsoVel), TorsoFlexionVelocity/1
  Inertia/1 -> CalcTorsoAcc/2, EndStops/3(TorsoInertia), TorsoSpring/3(TorsoInertia)
  Sum/1 -> Unit Delay/1
  CalcTorsoAcc/1 -> CalcTorsoVelocity/1
  Unit Delay/1 -> CalcTorsoAcc/1

== system LopesDevelopmentLibrary/Mindwalker/Mindwalker_Lopes_Conversion/VisualizeStickFigure ==
  TorsoFlexion : Inport
  Lopes_ModelPos : Inport  Port=2
  Enable : Inport  Port=3
  GetActuatedJoints : Selector  InputPortWidth=11  IndexOptions=Index vector (dialog)  Indices=1:8  OutputSizes=1
  Mux3 : Mux  Inputs=2
  Rate Transition : RateTransition
  Subsystem : Subsystem
  wires:
  Enable/1 -> Subsystem/Enable
  Rate Transition/1 -> Subsystem/1(In1)
  GetActuatedJoints/1 -> Mux3/1
  Lopes_ModelPos/1 -> GetActuatedJoints/1
  TorsoFlexion/1 -> Mux3/2
  Mux3/1 -> Rate Transition/1

== system LopesDevelopmentLibrary/Robot control blocks/FromLopes/GenerateString ==
  EnableAnaloginput : Inport
  Enable : EnablePort
  FromLopes_GenerateString : S-Function  InitFcn=try, set_param(gcb,'FunctionName','FromLopes_GenerateString'), end  FunctionName=FromLopes_GenerateString  SFunctionModules=FromLopes_GenerateString_wrapper  SFunctionDeploymentMode=off  EnableBusSupport=off  mask(S-Function Builder){}
      mask help: Simulink:masks:SFunctionBuilder_MD
      mask init: same as LopesDevelopmentLibrary/Various/SLRTMessage/S-Function Builder
      settings: CopyFcn=set_param(gcbh,'LinkStatus','none')  PreSaveFcn=try, set_param(gcb,'FunctionName','FromLopes_GenerateString'), end  OpenFcn=sfunctionwizard(gcbh)
      mask Display: plot(val(:,1),val(:,2)),disp(sys), port_label('input',1,'EnableAnalogInput'), port_label('output',1,'s'), port_label('output',2,'s_len')
  s : Outport
  s_len : Outport  Port=2
  wires:
  EnableAnaloginput/1 -> FromLopes_GenerateString/1
  FromLopes_GenerateString/1 -> s/1
  FromLopes_GenerateString/2 -> s_len/1

== system LopesDevelopmentLibrary/Robot control blocks/FromLopes/ParseString ==
  In1 : Inport
  In2 : Inport  Port=2
  Enable : EnablePort
  Data Type Conversion : DataTypeConversion  OutDataTypeStr=double
  FromLopes_ParseString : S-Function  InitFcn=try, set_param(gcb,'FunctionName','FromLopes_ParseString'), end  FunctionName=FromLopes_ParseString  SFunctionModules=FromLopes_ParseString_wrapper  SFunctionDeploymentMode=off  EnableBusSupport=off  mask(S-Function Builder){}
      mask help: Simulink:masks:SFunctionBuilder_MD
      mask init: same as LopesDevelopmentLibrary/Various/SLRTMessage/S-Function Builder
      settings: CopyFcn=set_param(gcbh,'LinkStatus','none')  PreSaveFcn=try, set_param(gcb,'FunctionName','FromLopes_ParseString'), end  OpenFcn=sfunctionwizard(gcbh)
      mask Display: plot(val(:,1),val(:,2)),disp(sys), port_label('input',1,'str'), port_label('input',2,'len'), port_label('output',1,'msgId'), port_label('output',2,'cnt'), port_label('output',3,'cntExpected'), port_label('output',4,'segmentModelPos'), port_label('output',5,'segmentModelVel'), port_label('output',6,'segmentModelAcc'), port_label('output',7,'segmentMeasPos'), port_label('output',8,'segmentMeasForce'), port_label('output',9,'cartesianModelPos'), port_label('output',10,'treadmill'), port_label('output',11,'analogInput')
  Logical Operator : Logic  Inputs=1  AllPortsSameDT=off  OutDataTypeStr=boolean
  MeasuredSegmentToAnatomicAngles : Subsystem
  MeasuredSegmentToAnatomicAngles1 : Subsystem
  MeasuredSegmentToAnatomicAngles2 : Subsystem
  MeasuredSegmentToAnatomicAngles3 : Subsystem
  MeasuredSegmentToAnatomicForce : Subsystem
  Relational Operator : RelationalOperator  Operator=~=  OutDataTypeStr=boolean
  Vector2CartesianPositionsBus : Subsystem
  cnt1 : Display  Commented=on
  cntExpected1 : Display  Commented=on
  msgID : Display  Commented=on
  ~Debug : Subsystem
      mask Display: disp('')
  ParseError : Outport
  ModelPos : Outport  Port=2
  ModelVel : Outport  Port=3
  ModelAcc : Outport  Port=4
  MeasPos : Outport  Port=5
  MeasForce : Outport  Port=6
  ModelCartPos : Outport  Port=7
  Treadmill : Outport  Port=8
  AnalogInput : Outport  Port=9
  wires:
  Logical Operator/1 -> Data Type Conversion/1
  FromLopes_ParseString/11 -> AnalogInput/1
  Data Type Conversion/1 -> ParseError/1
  FromLopes_ParseString/3 -> Relational Operator/2, cntExpected1/1
  FromLopes_ParseString/2 -> Relational Operator/1, cnt1/1
  FromLopes_ParseString/1 -> msgID/1
  FromLopes_ParseString/9 -> Vector2CartesianPositionsBus/1(In)
  In1/1 -> FromLopes_ParseString/1
  MeasuredSegmentToAnatomicAngles/1(Anatomic) -> ModelPos/1
  MeasuredSegmentToAnatomicAngles1/1(Anatomic) -> ModelVel/1
  FromLopes_ParseString/10 -> Treadmill/1
  Relational Operator/1 -> Logical Operator/1
  FromLopes_ParseString/8 -> MeasuredSegmentToAnatomicForce/1(segmentMeasForce)
  In2/1 -> FromLopes_ParseString/2
  FromLopes_ParseString/6 -> MeasuredSegmentToAnatomicAngles2/1(segmentModelX)
  FromLopes_ParseString/4 -> MeasuredSegmentToAnatomicAngles/1(segmentModelX)
  FromLopes_ParseString/5 -> MeasuredSegmentToAnatomicAngles1/1(segmentModelX)
  FromLopes_ParseString/7 -> MeasuredSegmentToAnatomicAngles3/1(segmentModelX)
  MeasuredSegmentToAnatomicAngles3/1(Anatomic) -> MeasPos/1
  Vector2CartesianPositionsBus/1(CartesianPositions) -> ModelCartPos/1
  MeasuredSegmentToAnatomicAngles2/1(Anatomic) -> ModelAcc/1
  MeasuredSegmentToAnatomicForce/1(AnatomicForce) -> MeasForce/1

== system LopesDevelopmentLibrary/Robot control blocks/FromLopes/~Debug ==

== system LopesDevelopmentLibrary/Robot control blocks/GeneralLopes/AnyMessageWasReceived ==
  In1 : Inport
  Compare To Constant : simulink/Logic and Bit Operations/Compare To Constant  relop=~=  const=-1  OutDataTypeStr=boolean
  Ground : Ground
  S-R Flip-Flop : simulink_extras/Flip Flops/S-R Flip-Flop  initial_condition=0
  Terminator : Terminator
  Out1 : Outport
  wires:
  Ground/1 -> S-R Flip-Flop/2
  S-R Flip-Flop/2 -> Terminator/1
  Compare To Constant/1 -> S-R Flip-Flop/1
  In1/1 -> Compare To Constant/1
  S-R Flip-Flop/1 -> Out1/1

== system LopesDevelopmentLibrary/Robot control blocks/GeneralLopes/GenerateString ==
  note: It appears that the first 100 (approx) messages are not
      | received by the LLC (does it take time to init the network card?)
      | We do want to initially set some values. I tried to do that at the
      | first message sent, but as that is not received, that doesn't work.
      | So, we just check whether we have received any message; if so,
      | we send the initializing stuff. This is what the AnyMessageWasReceived..
      | is for.
  DesiredState : Inport
  SegmentInertia : Inport  Port=2
  WatchdogTimeout_ms : Inport  Port=3
  AnyMessageWasReceivedByLLC : Inport  Port=4
  Enable : EnablePort
  Compare To Constant : simulink/Logic and Bit Operations/Compare To Constant  relop===  const=8  OutDataTypeStr=boolean
  Counter Free-Running : simulink/Sources/Counter Free-Running  NumBits=16  tsamp=-1
  Data Type Conversion1 : DataTypeConversion  OutDataTypeStr=double
  Detect Change : simulink/Logic and Bit Operations/Detect Change  vinit=0  InputProcessing=Inherited  OutDataTypeStr=boolean
  Detect Change1 : simulink/Logic and Bit Operations/Detect Change  vinit=nan  InputProcessing=Inherited  OutDataTypeStr=boolean
  Detect Change3 : simulink/Logic and Bit Operations/Detect Change  vinit=0  InputProcessing=Inherited  OutDataTypeStr=boolean
  Gain : Gain  Gain=ones(8,1)
  GeneralLopes_GenerateString : S-Function  InitFcn=try, set_param(gcb,'FunctionName','GeneralLopes_GenerateString'), end  FunctionName=GeneralLopes_GenerateString  SFunctionModules=GeneralLopes_GenerateString_wrapper  SFunctionDeploymentMode=off  EnableBusSupport=off  mask(S-Function Builder){}
      mask help: Simulink:masks:SFunctionBuilder_MD
      mask init: same as LopesDevelopmentLibrary/Various/SLRTMessage/S-Function Builder
      settings: CopyFcn=set_param(gcbh,'LinkStatus','none')  PreSaveFcn=try, set_param(gcb,'FunctionName','GeneralLopes_GenerateString'), end  OpenFcn=sfunctionwizard(gcbh)
      mask Display: plot(val(:,1),val(:,2)),disp(sys), port_label('input',1,'DesiredState'), port_label('input',2,'DesiredStateChanged'), port_label('input',3,'SegmentInertia'), port_label('input',4,'SegmentInertiaChanged'), port_label('input',5,'WatchdogTimeout'), port_label('input',6,'i'), port_label('output',1,'s'), port_label('output',2,'s_len')
  IsFirstSample : LopesDevelopmentLibrary/Various/IsFirstSample
  Logical Operator : Logic  Operator=OR  Inputs=1  AllPortsSameDT=off  OutDataTypeStr=boolean
  Logical Operator1 : Logic  AllPortsSameDT=off  OutDataTypeStr=boolean
  Logical Operator2 : Logic  Operator=NOT  AllPortsSameDT=off  OutDataTypeStr=boolean
  Logical Operator3 : Logic  AllPortsSameDT=off  OutDataTypeStr=boolean
  Logical Operator5 : Logic  Operator=OR  AllPortsSameDT=off  OutDataTypeStr=boolean
  Rounding Function : Rounding
  Width : Width
  s : Outport
  s_len : Outport  Port=2
  wires:
  Rounding Function/1 -> GeneralLopes_GenerateString/1
  Logical Operator5/1 -> Logical Operator1/1
  Detect Change3/1 -> Logical Operator5/2
  AnyMessageWasReceivedByLLC/1 -> Detect Change3/1
  Data Type Conversion1/1 -> GeneralLopes_GenerateString/6
  Counter Free-Running/1 -> Data Type Conversion1/1
  Logical Operator2/1 -> Logical Operator3/1
  IsFirstSample/1 -> Logical Operator2/1
  Logical Operator3/1 -> GeneralLopes_GenerateString/2
  Logical Operator1/1 -> GeneralLopes_GenerateString/4
  Logical Operator/1 -> Logical Operator5/1
  Compare To Constant/1 -> Logical Operator1/2
  Width/1 -> Compare To Constant/1
  SegmentInertia/1 -> Gain/1, Width/1
  Gain/1 -> Detect Change1/1, GeneralLopes_GenerateString/3
  Detect Change1/1 -> Logical Operator/1
  Detect Change/1 -> Logical Operator3/2
  GeneralLopes_GenerateString/1 -> s/1
  DesiredState/1 -> Rounding Function/1, Detect Change/1
  GeneralLopes_GenerateString/2 -> s_len/1
  WatchdogTimeout_ms/1 -> GeneralLopes_GenerateString/5

== system LopesDevelopmentLibrary/Robot control blocks/GeneralLopes/ParseString ==
  s : Inport
  s_len : Inport  Port=2
  Enable : EnablePort
  GeneralLopes_ParseString : S-Function  InitFcn=try, set_param(gcb,'FunctionName','GeneralLopes_ParseString'), end  FunctionName=GeneralLopes_ParseString  SFunctionModules=GeneralLopes_ParseString_wrapper  SFunctionDeploymentMode=off  EnableBusSupport=off  mask(S-Function Builder){}
      mask help: Simulink:masks:SFunctionBuilder_MD
      mask init: same as LopesDevelopmentLibrary/Various/SLRTMessage/S-Function Builder
      settings: CopyFcn=set_param(gcbh,'LinkStatus','none')  PreSaveFcn=try, set_param(gcb,'FunctionName','GeneralLopes_ParseString'), end  OpenFcn=sfunctionwizard(gcbh)
      mask Display: plot(val(:,1),val(:,2)),disp(sys), port_label('input',1,'s'), port_label('input',2,'s_len'), port_label('output',1,'isParseException'), port_label('output',2,'llcState'), port_label('output',3,'blueCabinetButtonPressed'), port_label('output',4,'isInitOk'), port_label('output',5,'isMotorsOk'), port_label('output',6,'isTreadmillEmpty'), port_label('output',7,'isPatientDefined')
  isParseException : Outport  InitialOutput=[-1]
  llcState : Outport  Port=2
  isBlueCabinetButtonPressed : Outport  Port=3
  isInitOk : Outport  Port=4
  isMotorsOk : Outport  Port=5
  isTreadmillEmpty : Outport  Port=6
  isPatientDefined : Outport  Port=7
  wires:
  GeneralLopes_ParseString/7 -> isPatientDefined/1  "isPatientDefined"
  GeneralLopes_ParseString/3 -> isBlueCabinetButtonPressed/1  "isCabinetBlueButtonPressed"
  GeneralLopes_ParseString/2 -> llcState/1  "llcState"
  GeneralLopes_ParseString/6 -> isTreadmillEmpty/1  "isTreadmillEmpty"
  GeneralLopes_ParseString/4 -> isInitOk/1  "isInitOk"
  GeneralLopes_ParseString/5 -> isMotorsOk/1  "isMotorsOk"
  s_len/1 -> GeneralLopes_ParseString/2
  s/1 -> GeneralLopes_ParseString/1
  GeneralLopes_ParseString/1 -> isParseException/1

== system LopesDevelopmentLibrary/Robot control blocks/GeneralLopes/~Debug ==

== system LopesDevelopmentLibrary/Robot control blocks/ToLopes/CrossFade ==
  In1 : Inport
  In2 : Inport  Port=2
  AmountIn2 : Inport  Port=3
  Add : Sum  Inputs=+-
  Add1 : Sum
  One : Constant
  Product : Product  RndMeth=Zero
  Product1 : Product  RndMeth=Zero
  Saturation : Saturate  UpperLimit=1  LowerLimit=0
  Out : Outport
  wires:
  Add1/1 -> Out/1
  In2/1 -> Product/1
  Product1/1 -> Add1/1
  Product/1 -> Add1/2
  Add/1 -> Product1/2
  Saturation/1 -> Add/2, Product/2
  One/1 -> Add/1
  AmountIn2/1 -> Saturation/1
  In1/1 -> Product1/1

== system LopesDevelopmentLibrary/Robot control blocks/ToLopes/CrossFade1 ==
  In1 : Inport
  In2 : Inport  Port=2
  AmountIn2 : Inport  Port=3
  Add : Sum  Inputs=+-
  Add1 : Sum
  One : Constant
  Product : Product  RndMeth=Zero
  Product1 : Product  RndMeth=Zero
  Saturation : Saturate  UpperLimit=1  LowerLimit=0
  Out : Outport
  wires:
  In1/1 -> Product1/1
  AmountIn2/1 -> Saturation/1
  One/1 -> Add/1
  Saturation/1 -> Product/2, Add/2
  Add/1 -> Product1/2
  Product/1 -> Add1/2
  Product1/1 -> Add1/1
  In2/1 -> Product/1
  Add1/1 -> Out/1
